simulink subsystem "Main_Contactor_Closed"  (R2023b)
settings: Solver=VariableStepAuto  StartTime=0.0  StopTime=10.0  RelTol=1e-3
settings Model: Creator=diego  LastModifiedBy=diego

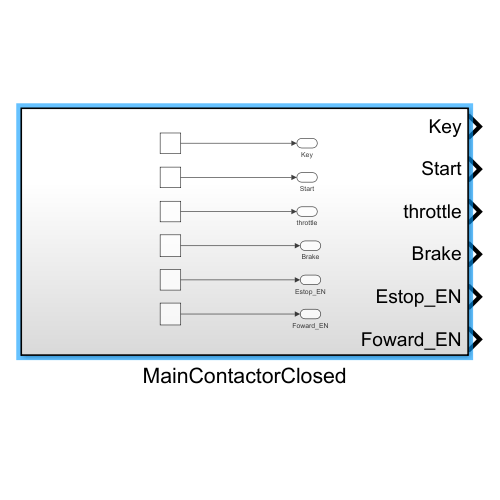
[thumbnail: Simulink's stored preview of the top-level diagram]
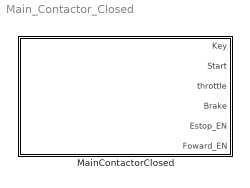
== system Main_Contactor_Closed ==
  MainContactorClosed : Subsystem

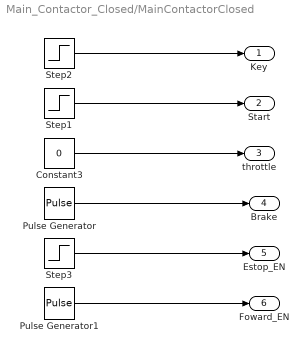
== system Main_Contactor_Closed/MainContactorClosed ==
  Constant3 : Constant  Value=0
  Pulse Generator : DiscretePulseGenerator  PulseType=Time based  Period=100  PulseWidth=50
  Pulse Generator1 : DiscretePulseGenerator  PulseType=Time based  Period=100  PulseWidth=50
  Step1 : Step  Time=300  SampleTime=0
  Step2 : Step  Time=100  SampleTime=0
  Step3 : Step  Time=400  SampleTime=0
  Key : Outport
  Start : Outport  Port=2
  throttle : Outport  Port=3
  Brake : Outport  Port=4
  Estop_EN : Outport  Port=5
  Foward_EN : Outport  Port=6
  wires:
  Step2/1 -> Key/1
  Step1/1 -> Start/1
  Constant3/1 -> throttle/1
  Pulse Generator/1 -> Brake/1
  Step3/1 -> Estop_EN/1
  Pulse Generator1/1 -> Foward_EN/1
